simulink model "q11"  (R2017b)
settings: Solver=VariableStepAuto  StartTime=0.0  StopTime=5  RelTol=1e-3
undefined symbols (not defined in the file): Az, Bz, Cz, K
libraries: peLuenbergerObserver x1
settings Model: Creator=admin  LastModifiedBy=admin

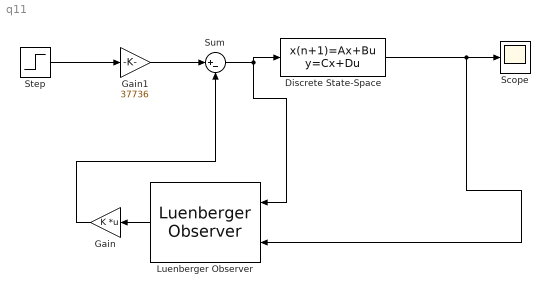
== system q11 ==
  Discrete State-Space : DiscreteStateSpace  A=Az  B=Bz  C=Cz  D=[0]  SampleTime=0.004
  Gain : Gain  Gain=K  Multiplication=Matrix(K*u)
  Gain1 : Gain  Gain=37736
  Luenberger Observer : peLuenbergerObserver/Luenberger Observer  StateSpaceType=Discrete-time  Ad=Az  Bd=Bz  Cd=Cz  Dd=Dz  A=1  B=1  C=1  D=1  ObserverDesign=Observer gain  Ld=L  DesiredEigenvalues=0  x0=[0 ;0; 0]  Tsd=0.1  Ts=0.004
  Scope : Scope
  Step : Step  SampleTime=0
  Sum : Sum  Inputs=|+-
  wires:
  Gain/1 -> Sum/2
  Discrete State-Space/1 -> Luenberger Observer/2, Scope/1
  Sum/1 -> Discrete State-Space/1, Luenberger Observer/1
  Luenberger Observer/1 -> Gain/1
  Gain1/1 -> Sum/1
  Step/1 -> Gain1/1
